simulink model "symulacja_1_9_p2"  (R2019b)
settings: Solver=VariableStepAuto  StartTime=0  StopTime=8000  FixedStep=1  MaxStep=1.5  MinStep=0.5  RelTol=1
undefined symbols (not defined in the file or in its folder): sigbuilder_block
libraries: simulink x3
settings Model: SimulationMode=accelerator  Creator=kuba9  LastModifiedBy=ny9a
settings SolverCC: InitialStep=1

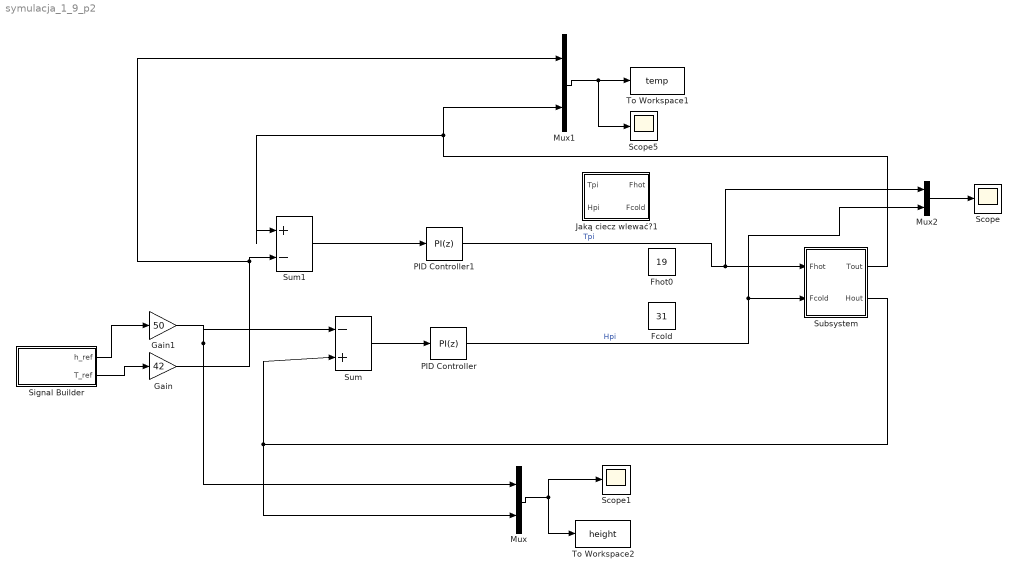
== system symulacja_1_9_p2 ==
  "Fcold " : Constant  Value=31
  "Fhot0 " : Constant  Value=19
  Gain : Gain  Gain=42
  Gain1 : Gain  Gain=50
  Jaką ciecz wlewać?1 : Subsystem
  Mux : Mux  Inputs=2
  Mux1 : Mux  Inputs=2
  Mux2 : Mux  Inputs=2
  PID Controller : simulink/Continuous/PID Controller  Controller=PI  Form=Ideal  TimeDomain=Discrete-time  SampleTime=-1  IntegratorMethod=Backward Euler  FilterMethod=Forward Euler  ControllerParametersSource=internal  P=-3000  I=1  D=1.52211780745286  UseFilter=off  N=100  TunerSelectOption=Transfer Function Based (PID Tuner App)  ZeroCross=off  InitialConditionSource=internal  InitialConditionForIntegrator=38  InitialConditionForFilter=0  DifferentiatorICPrevScaledInput=50  ExternalReset=none  TrackingMode=off  Kt=1  LimitOutput=on  UpperSaturationLimit=inf  LowerSaturationLimit=0  LinearizeAsGain=off  AntiWindupMode=none  Kb=1  POutMin=[]  POutMax=[]  IOutMin=[]  IOutMax=[]  DOutMin=[]  DOutMax=[]  NOutMin=[]  NOutMax=[]  SumOutMin=[]  SumOutMax=[]  SaturationOutMin=[]  SaturationOutMax=[]  PParamMin=[]  PParamMax=[]  IParamMin=[]  IParamMax=[]  DParamMin=[]  DParamMax=[]  NParamMin=[]  NParamMax=[]  KbParamMin=[]  KbParamMax=[]  KtParamMin=[]  KtParamMax=[]  KbOutMin=[]  KbOutMax=[]  KtOutMin=[]  KtOutMax=[]  IntegratorOutMin=[]  IntegratorOutMax=[]  FilterOutMin=[]  FilterOutMax=[]  SumI1OutMin=[]  SumI1OutMax=[]  SumI2OutMin=[]  SumI2OutMax=[]  SumI3OutMin=[]  SumI3OutMax=[]  SumI4OutMin=[]  SumI4OutMax=[]  SumDOutMin=[]  SumDOutMax=[]  DifferentiatorOutMin=[]  DifferentiatorOutMax=[]  FilterDiffOutCoefMin=[]  FilterDiffOutCoefMax=[]  ReciprocalOutMin=[]  ReciprocalOutMax=[]  SumDenOutMin=[]  SumDenOutMax=[]  SumNumOutMin=[]  SumNumOutMax=[]  DivideOutMin=[]  DivideOutMax=[]  IntegratorContinuousStateAttributes=''  IntegratorStateMustResolveToSignalObject=off  IntegratorRTWStateStorageClass=Auto  FilterContinuousStateAttributes=''  FilterStateMustResolveToSignalObject=off  FilterRTWStateStorageClass=Auto  ParallelPVariant=Passthrough  IdealPVariant=InternalParameters  IVariant=InternalParameters  DVariant=Disabled  IntegratorVariant=Discrete  SatVariant=Enabled  AWVariant=Passthrough  PCopyVariant=Disabled  TRVariant=Disabled  FdbkBlocksVariant=Forward  IdealPFdbkVariant=Disabled  SatFdbkVariant=Disabled  DerivativeFilterVariant=Disabled  NVariant=Disabled  NCopyVariant=Disabled_SignalSpec  FilterICVariant=Disabled  IntegratorICVariant=InternalICs  ExternalResetVariant=Disabled  TRSumVariant=Passthrough  SumFdbkVariant=Disabled  SumVariant=Sum_PI
  PID Controller1 : simulink/Continuous/PID Controller  Controller=PI  Form=Parallel  TimeDomain=Discrete-time  SampleTime=-1  IntegratorMethod=Backward Euler  FilterMethod=Forward Euler  ControllerParametersSource=internal  P=-527.810549971366  I=-70.0719974691964  D=5  UseFilter=on  N=100  TunerSelectOption=Transfer Function Based (PID Tuner App)  ZeroCross=off  InitialConditionSource=internal  InitialConditionForIntegrator=0  InitialConditionForFilter=0  DifferentiatorICPrevScaledInput=0  ExternalReset=none  TrackingMode=off  Kt=1  LimitOutput=on  UpperSaturationLimit=inf  LowerSaturationLimit=0  LinearizeAsGain=on  AntiWindupMode=none  Kb=1  POutMin=[]  POutMax=[]  IOutMin=[]  IOutMax=[]  DOutMin=[]  DOutMax=[]  NOutMin=[]  NOutMax=[]  SumOutMin=[]  SumOutMax=[]  SaturationOutMin=[]  SaturationOutMax=[]  PParamMin=[]  PParamMax=[]  IParamMin=[]  IParamMax=[]  DParamMin=[]  DParamMax=[]  NParamMin=[]  NParamMax=[]  KbParamMin=[]  KbParamMax=[]  KtParamMin=[]  KtParamMax=[]  KbOutMin=[]  KbOutMax=[]  KtOutMin=[]  KtOutMax=[]  IntegratorOutMin=[]  IntegratorOutMax=[]  FilterOutMin=[]  FilterOutMax=[]  SumI1OutMin=[]  SumI1OutMax=[]  SumI2OutMin=[]  SumI2OutMax=[]  SumI3OutMin=[]  SumI3OutMax=[]  SumI4OutMin=[]  SumI4OutMax=[]  SumDOutMin=[]  SumDOutMax=[]  DifferentiatorOutMin=[]  DifferentiatorOutMax=[]  FilterDiffOutCoefMin=[]  FilterDiffOutCoefMax=[]  ReciprocalOutMin=[]  ReciprocalOutMax=[]  SumDenOutMin=[]  SumDenOutMax=[]  SumNumOutMin=[]  SumNumOutMax=[]  DivideOutMin=[]  DivideOutMax=[]  IntegratorContinuousStateAttributes=''  IntegratorStateMustResolveToSignalObject=off  IntegratorRTWStateStorageClass=Auto  FilterContinuousStateAttributes=''  FilterStateMustResolveToSignalObject=off  FilterRTWStateStorageClass=Auto  ParallelPVariant=InternalParameters  IdealPVariant=Disabled  IVariant=InternalParameters  DVariant=Disabled  IntegratorVariant=Discrete  SatVariant=Enabled  AWVariant=Passthrough  PCopyVariant=Disabled  TRVariant=Disabled  FdbkBlocksVariant=Forward  IdealPFdbkVariant=Disabled  SatFdbkVariant=Disabled  DerivativeFilterVariant=Disabled  NVariant=Disabled  NCopyVariant=Disabled_SignalSpec  FilterICVariant=Disabled  IntegratorICVariant=InternalICs  ExternalResetVariant=Disabled  TRSumVariant=Passthrough  SumFdbkVariant=Disabled  SumVariant=Sum_PI
  Scope : Scope
  Scope1 : Scope
  Scope5 : Scope
  Signal Builder : Subsystem  Tag=STV Subsys  LoadFcn=sigbuilder_block('load');  StartFcn=sigbuilder_block('start');  StopFcn=sigbuilder_block('stop');  ClipboardFcn=sigbuilder_block('clipboard');  mask(Sigbuilder block){tuvar=[0:10]}
      mask help: Simulink:masks:SigbuilderBlock_MD
      mask init:
      | if ~strcmp(get_param(bdroot(gcbh),'SimulationStatus'),'stopped') tuvar = sigbuilder_block('maskInit'); end
      settings: CopyFcn=sigbuilder_block('copy');  DeleteFcn=sigbuilder_block('delete');  ModelCloseFcn=sigbuilder_block('modelClose');  PreSaveFcn=sigbuilder_block('preSave');  PauseFcn=sigbuilder_block('pause');  ContinueFcn=sigbuilder_block('continue');  NameChangeFcn=sigbuilder_block('namechange');  OpenFcn=sigbuilder_block('open',[6 30 1012.5 447.75 ]);  CloseFcn=sigbuilder_block('close');
      mask Display: plot(0, 0, 100, 100,[2, 2, 32, 32, 2], [68, 8, 8, 68, 68],[32, 2], [38, 38], [32, 19, 2],[53, 60, 44], [32, 17, 17, 2],[16, 16, 31, 31]);txt = getActiveGroup(gcbh);text(2, 100, txt,'verticalAlignment', 'top');
  Subsystem : Subsystem
  Sum : Sum  Inputs=|-+
  Sum1 : Sum  Inputs=|+-
  To Workspace1 : ToWorkspace  VariableName=temp  SaveFormat=Structure  SampleTime=-1
      settings: Save2DSignal=2-D array (concatenate along first dimension)
  To Workspace2 : ToWorkspace  VariableName=height  SaveFormat=Structure  SampleTime=-1
      settings: Save2DSignal=2-D array (concatenate along first dimension)
  wires:
  Signal Builder/1(h_ref) -> Gain1/1
  Signal Builder/2(T_ref) -> Gain/1
  Mux1/1 -> To Workspace1/1, Scope5/1
  Sum/1 -> PID Controller/1
  Gain1/1 -> Mux/1, Sum/1
  Mux/1 -> Scope1/1, To Workspace2/1
  Mux2/1 -> Scope/1
  Subsystem/2(Hout) -> Sum/2, Mux/2
  Subsystem/1(Tout) -> Mux1/2, Sum1/1
  PID Controller/1 -> Subsystem/2("Fcold "), Mux2/2  "Hpi"
  Sum1/1 -> PID Controller1/1
  Gain/1 -> Mux1/1, Sum1/2
  PID Controller1/1 -> Mux2/1, Subsystem/1("Fhot ")  "Tpi"

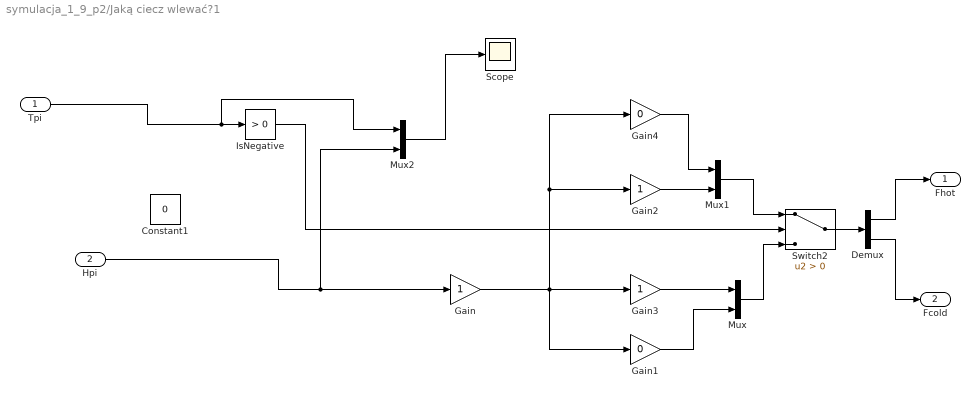
== system symulacja_1_9_p2/Jaką ciecz wlewać?1 ==
  Tpi : Inport
  Hpi : Inport  Port=2
  Constant1 : Constant  Value=0
  Demux : Demux  Outputs=2
  Gain : Gain
  Gain1 : Gain  Gain=0
  Gain2 : Gain
  Gain3 : Gain
  Gain4 : Gain  Gain=0
  IsNegative : simulink/Logic and Bit Operations/Compare To Zero  relop=>  OutDataTypeStr=boolean  ZeroCross=off
  Mux : Mux  Inputs=2
  Mux1 : Mux  Inputs=2
  Mux2 : Mux  Inputs=2
  Scope : Scope
  Switch2 : Switch  Criteria=u2 > Threshold
  Fhot : Outport
  Fcold : Outport  Port=2
  wires:
  Tpi/1 -> IsNegative/1, Mux2/1
  Mux2/1 -> Scope/1
  Hpi/1 -> Gain/1, Mux2/2
  Gain/1 -> Gain3/1, Gain1/1, Gain2/1, Gain4/1
  IsNegative/1 -> Switch2/2
  Demux/2 -> Fcold/1
  Demux/1 -> Fhot/1
  Switch2/1 -> Demux/1
  Mux/1 -> Switch2/3
  Mux1/1 -> Switch2/1
  Gain4/1 -> Mux1/1
  Gain2/1 -> Mux1/2
  Gain1/1 -> Mux/2
  Gain3/1 -> Mux/1

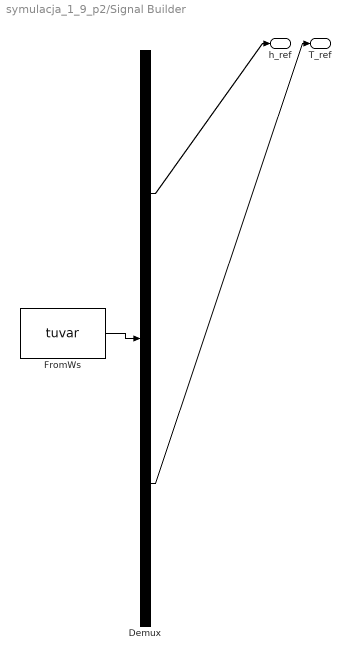
== system symulacja_1_9_p2/Signal Builder ==
  Demux : Demux  Tag=STV Demux  Outputs=2
  FromWs : FromWorkspace  Tag=STV FromWs  VariableName=tuvar  SampleTime=0
      SigBuilderData=|
      | common.afterFinalStr = 'Extrapolate'
      | common.sampleTime = 0
      | dataSet.timeRange = [0 8000]
      | dataSet.name = 'Group 1'
      | sbobj.Groups.Name = 'Group 1'
      | sbobj.Groups.Signals(1).Name = 'h_ref'
      | sbobj.Groups.Signals(1).XData = [0 1000 1100 3100 3600 8000]
      | sbobj.Groups.Signals(1).YData = [1 1 1.2 1.2 1 1]
      | sbobj.Groups.Signals(2).Name = 'T_ref'
      | sbobj.Groups.Signals(2).XData = [0 2000 3000 4460 5000 6000 8000]
      | sbobj.Groups.Signals(2).YData = [1 1 0.8 0.8 0.8 0.7 0.7]
      | sbobj.Groups.TimeRange = [0 8000]
  h_ref : Outport  Tag=STV Outport
  T_ref : Outport  Tag=STV Outport  Port=2
  wires:
  FromWs/1 -> Demux/1
  Demux/1 -> h_ref/1
  Demux/2 -> T_ref/1

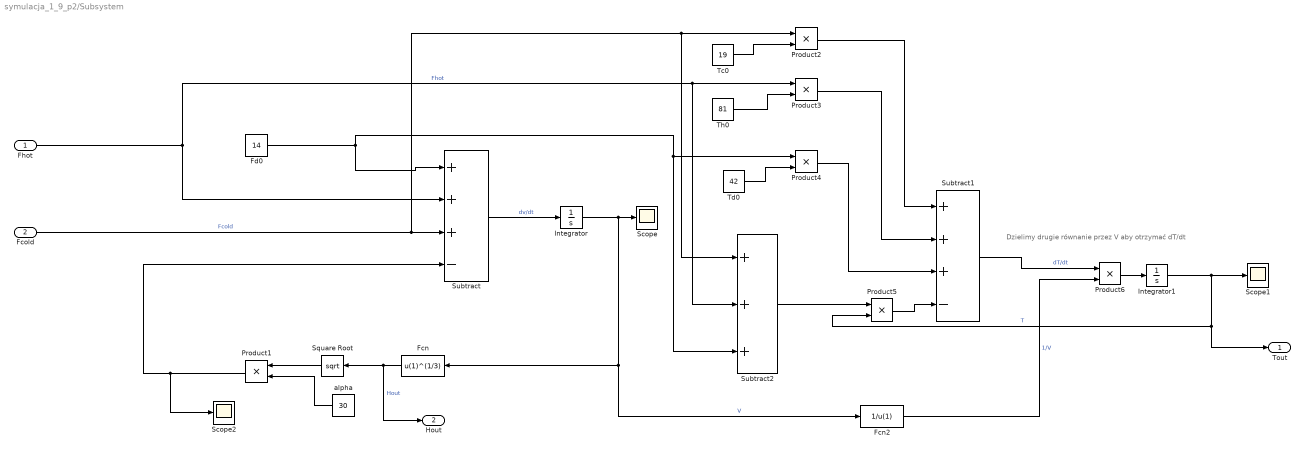
== system symulacja_1_9_p2/Subsystem ==
  note: Dzielimy drugie równanie przez V aby otrzymać dT/dt
  "Fhot " : Inport
  "Fcold " : Inport  Port=2
  Fcn : Fcn  Expr=u(1)^(1/3)
  Fcn2 : Fcn  Expr=1/u(1)
  Fd0 : Constant  Value=14
  Integrator : Integrator  InitialCondition=125000  ZeroCross=off
  Integrator1 : Integrator  InitialCondition=42
  Product{1..6} (6 alike) : Product
  Scope : Scope
  Scope1 : Scope
  Scope2 : Scope
  Square Root : Sqrt  SaturateOnIntegerOverflow=on
  Subtract : Sum  Inputs=+++-
  Subtract1 : Sum  Inputs=+++-
  Subtract2 : Sum  Inputs=+++
  Tc0 : Constant  Value=19
  Td0 : Constant  Value=42
  Th0 : Constant  Value=81
  alpha : Constant  Value=30
  Tout : Outport
  Hout : Outport  Port=2
  wires:
  "Fcold "/1 -> Subtract2/1, Product2/1, Subtract/3  "Fcold"
  Integrator/1 -> Fcn/1, Fcn2/1, Scope/1  "V"
  alpha/1 -> Product1/2
  Fd0/1 -> Subtract/1, Subtract2/3, Product4/1
  Th0/1 -> Product3/2
  Td0/1 -> Product4/2
  Product2/1 -> Subtract1/1
  Fcn/1 -> Hout/1, Square Root/1  "Hout"
  "Fhot "/1 -> Subtract/2, Subtract2/2, Product3/1  "Fhot"
  Tc0/1 -> Product2/2
  Integrator1/1 -> Product5/2, Tout/1, Scope1/1  "T"
  Subtract/1 -> Integrator/1  "dv/dt"
  Subtract1/1 -> Product6/1  "dT/dt"
  Product4/1 -> Subtract1/3
  Subtract2/1 -> Product5/1
  Product6/1 -> Integrator1/1
  Product3/1 -> Subtract1/2
  Product5/1 -> Subtract1/4
  Fcn2/1 -> Product6/2  "1/V"
  Square Root/1 -> Product1/1
  Product1/1 -> Scope2/1, Subtract/4
